simulink model "importance_resampling"  (R2021b)
settings: Solver=VariableStepAuto  StartTime=0.0  StopTime=100  RelTol=1e-3
libraries: wnnlib x2
settings Model: Creator=20214358  LastModifiedBy=20214358

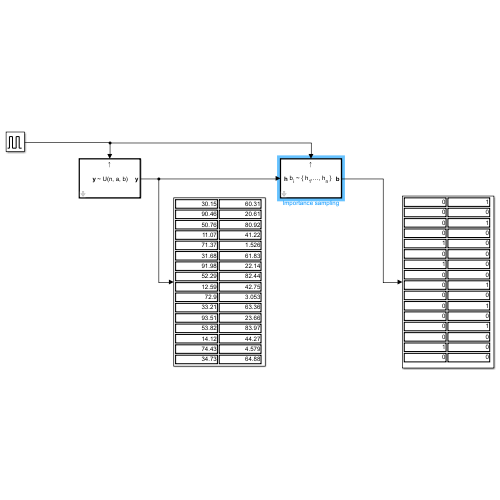
[thumbnail: Simulink's stored preview of the top-level diagram]
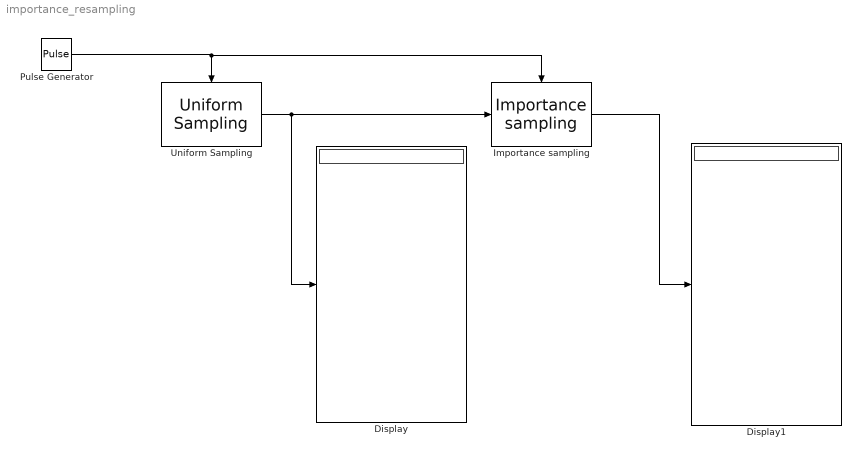
== system importance_resampling ==
  Display : Display
  Display1 : Display
  Importance sampling : wnnlib/Utilities/Importance sampling  nSamples=8
      settings: SourceProductName=Weightless Neural Networks Toolbox
  Pulse Generator : DiscretePulseGenerator  PulseType=Time based  Period=1  PulseWidth=5
  Uniform Sampling : wnnlib/Sources/Uniform Sampling  nSamples=32  min_value=0  max_value=100  nSeed=0
      settings: SourceProductName=Weightless Neural Networks Toolbox
  wires:
  Uniform Sampling/1 -> Display/1, Importance sampling/1
  Pulse Generator/1 -> Importance sampling/Trigger, Uniform Sampling/Trigger
  Importance sampling/1 -> Display1/1
